simulink model "simuV6_restored_from_autosave"  (R2016a)
settings: Solver=VariableStepAuto  StartTime=0.0  StopTime=20  RelTol=1e-3
libraries: powerlib x15, powerlib_meascontrol x2, simulink x1
settings Model: Creator=EEE  LastModifiedBy=mbonea godwin

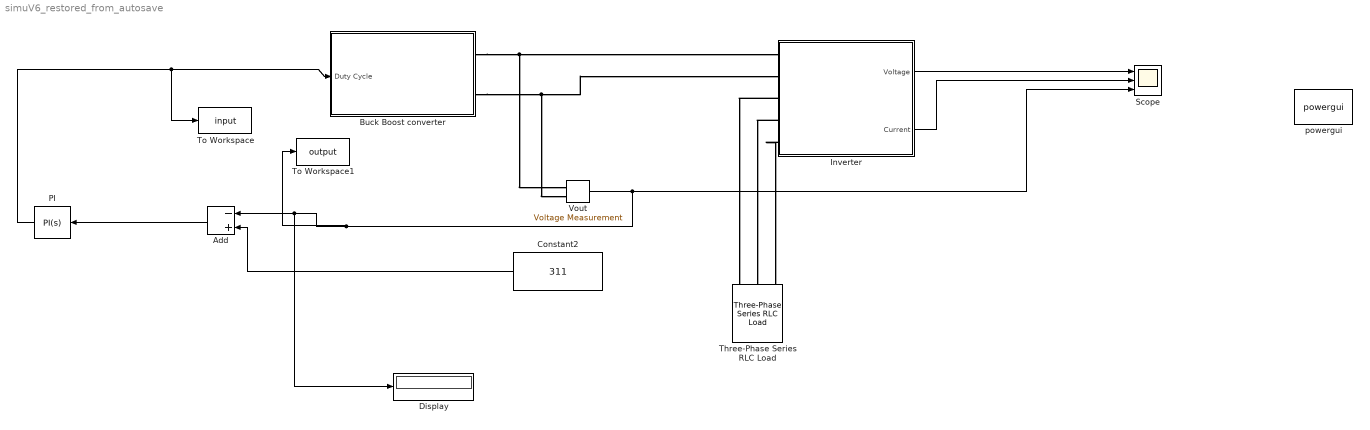
== system simuV6_restored_from_autosave ==
  Add : Sum  Inputs=-+
  Buck Boost converter : Subsystem
  Constant2 : Constant  Value=311
  Display : Display
  Inverter : Subsystem
  PI : simulink/Continuous/PID Controller  Controller=PI  TimeDomain=Continuous-time  SampleTime=-1  IntegratorMethod=Forward Euler  FilterMethod=Forward Euler  Form=Parallel  UseFilter=on  ControllerParametersSource=internal  P=43.0737287073608  I=6.97946285462644  D=0  N=100  InitialConditionSource=internal  InitialConditionForIntegrator=0  InitialConditionForFilter=0  ExternalReset=none  LimitOutput=on  UpperSaturationLimit=0.9  LowerSaturationLimit=0.1  LinearizeAsGain=on  AntiWindupMode=none  Kb=1  TrackingMode=off  Kt=1  PParamMin=[]  PParamMax=[]  IParamMin=[]  IParamMax=[]  DParamMin=[]  DParamMax=[]  NParamMin=[]  NParamMax=[]  KbParamMin=[]  KbParamMax=[]  KtParamMin=[]  KtParamMax=[]  POutMin=[]  POutMax=[]  IOutMin=[]  IOutMax=[]  DOutMin=[]  DOutMax=[]  NOutMin=[]  NOutMax=[]  KbOutMin=[]  KbOutMax=[]  KtOutMin=[]  KtOutMax=[]  IntegratorOutMin=[]  IntegratorOutMax=[]  FilterOutMin=[]  FilterOutMax=[]  SumOutMin=[]  SumOutMax=[]  SumI1OutMin=[]  SumI1OutMax=[]  SumI2OutMin=[]  SumI2OutMax=[]  SumI3OutMin=[]  SumI3OutMax=[]  SumDOutMin=[]  SumDOutMax=[]  SaturationOutMin=[]  SaturationOutMax=[]  IntegratorContinuousStateAttributes=''  IntegratorStateMustResolveToSignalObject=off  IntegratorRTWStateStorageClass=Auto  FilterContinuousStateAttributes=''  FilterStateMustResolveToSignalObject=off  FilterRTWStateStorageClass=Auto  DifferentiatorICPrevScaledInput=0  DifferentiatorOutMin=[]  DifferentiatorOutMax=[]
  Scope : Scope  NumInputPorts=3
  Three-Phase Series RLC Load : powerlib/Elements/Three-Phase Series RLC Load  LConnTagsString=A|B|C  Configuration=Y (grounded)  NominalVoltage=220  Vabc=[1e3 1e3 1e3]  Vabcp=[1e3 1e3 1e3]  NominalFrequency=50  UnbalancedPower=off  ActivePower=10e3  InductivePower=0  CapacitivePower=0  Pabc=[10e3 9e3 11e3]  QLabc=[100 90 110]  QCabc=[100 90 110]  Pabcp=[10e3 9e3 11e3]  QLabcp=[100 90 110]  QCabcp=[100 90 110]  Measurements=None  LoadType=constant Z
  To Workspace : ToWorkspace  VariableName=input  SaveFormat=Timeseries  SampleTime=-1
  To Workspace1 : ToWorkspace  VariableName=output  SaveFormat=Timeseries  SampleTime=-1
  Vout : powerlib/Measurements/Voltage Measurement  PhasorSimulation=off  OutputType=Complex  PSBequivalent=0
  powergui : powerlib/powergui  Priority=1  SimulationMode=Continuous  SolverType=Tustin/Backward Euler (TBE)  SampleTime=50e-6  frequency=60  SPID=on  DisableSnubberDevices=off  DisableRonSwitches=off  DisableVfSwitches=off  SwTol=0  DisplayEquations=off  Interpol=off  ExternalGateDelay=off  methode=off  Ts=10  FunctionMessages=off  echomessages=off  HookPort=off  EnableUseOfTLC=off  x0status=blocks  frequencyindice=0  Pbase=100e6  ErrMax=1e-4  Iterations=50  UnitsV=kV  UnitsW=MW  buscounter=0  RestoreLinks=warning  ResistiveCurrentMeasurement=off  Frange=[0:2:500]  Ylog=off  Xlog=on  ShowGrid=off  save=off  variable=ZData  structure=0  ZoomFFT=off  StartTime=0.0  cycles=1  DisplayStyle=1  fundamental=60  FreqAxis=off  MaxFrequency=1000  frequencyindicesteady=1  RmsSteady=1  display=off
  wires:
  Vout/1 -> To Workspace1/1, Display/1, Add/1, Scope/3
  Inverter/2(Current) -> Scope/2
  Inverter/1(Voltage) -> Scope/1
  Constant2/1 -> Add/2
  Add/1 -> PI/1
  PI/1 -> To Workspace/1, Buck Boost converter/1(Duty Cycle)
  connections:
  Buck Boost converter/RConn1 -- Vout/LConn1 -- Inverter/LConn1
  Buck Boost converter/RConn2 -- Vout/LConn2 -- Inverter/LConn2
  Inverter/LConn5 -- Three-Phase Series RLC Load/LConn3
  Inverter/LConn4 -- Three-Phase Series RLC Load/LConn2
  Inverter/LConn3 -- Three-Phase Series RLC Load/LConn1

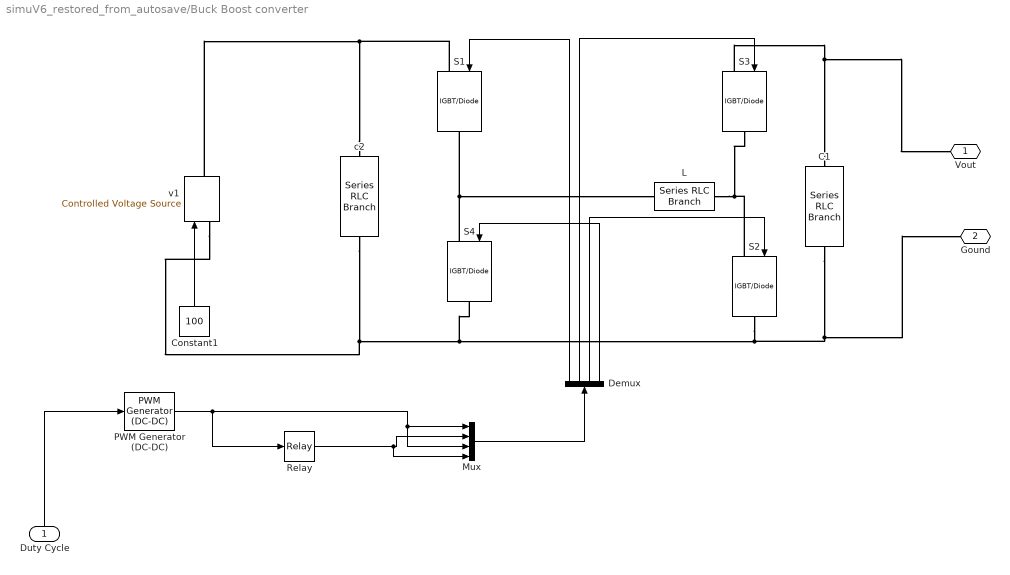
== system simuV6_restored_from_autosave/Buck Boost converter ==
  Duty Cycle : Inport
  "C1 " : powerlib/Elements/Series RLC Branch  LConnTagsString=__new0  RConnTagsString=__new0  BranchType=C  Resistance=1  Inductance=1e-3  SetiL0=off  InitialCurrent=0  Capacitance=20000000e-6  Setx0=off  InitialVoltage=0  Measurements=None
  Constant1 : Constant  Value=100
  Demux : Demux
  "L " : powerlib/Elements/Series RLC Branch  LConnTagsString=__new0  RConnTagsString=__new0  BranchType=L  Resistance=1  Inductance=1e-4  SetiL0=off  InitialCurrent=0  Capacitance=20000e-6  Setx0=off  InitialVoltage=0  Measurements=Branch voltage and current
  Mux : Mux
  PWM Generator (DC-DC) : powerlib_meascontrol/Pulse & Signal Generators/PWM Generator (DC-DC)  Fsw=5000  Ts=0
  Relay : Relay  OnOutputValue=0  OffOutputValue=1
  S{1..4} (4 alike) : powerlib/Power Electronics/IGBT//Diode  Ron=1e-3  Rs=1e5  Cs=inf  Measurements=off
  "c2 " : powerlib/Elements/Series RLC Branch  LConnTagsString=__new0  RConnTagsString=__new0  BranchType=RC  Resistance=10  Inductance=1e-3  SetiL0=off  InitialCurrent=0  Capacitance=15000e-6  Setx0=off  InitialVoltage=0  Measurements=None
  "v1 " : powerlib/Electrical Sources/Controlled Voltage Source  Initialize=on  Source_Type=DC  Amplitude=0  Phase=0  Frequency=0  Measurements=None
  Vout : PMIOPort  Port=1  Side=Right
  Gound : PMIOPort  Port=2  Side=Right
  wires:
  Duty Cycle/1 -> PWM Generator (DC-DC)/1
  Demux/2 -> S3/1
  Mux/1 -> Demux/1
  Demux/3 -> S2/1
  PWM Generator (DC-DC)/1 -> Relay/1, Mux/3, Mux/1
  Demux/4 -> S4/1
  Relay/1 -> Mux/4, Mux/2
  Constant1/1 -> "v1 "/1
  Demux/1 -> S1/1
  connections:
  S3/RConn1 -- "L "/LConn1 -- S2/LConn1
  S1/RConn1 -- "L "/RConn1 -- S4/LConn1
  S2/RConn1 -- Gound/RConn1 -- "C1 "/RConn1 -- S4/RConn1 -- "c2 "/RConn1 -- "v1 "/LConn1
  S3/LConn1 -- Vout/RConn1 -- "C1 "/LConn1
  "c2 "/LConn1 -- "v1 "/RConn1 -- S1/LConn1

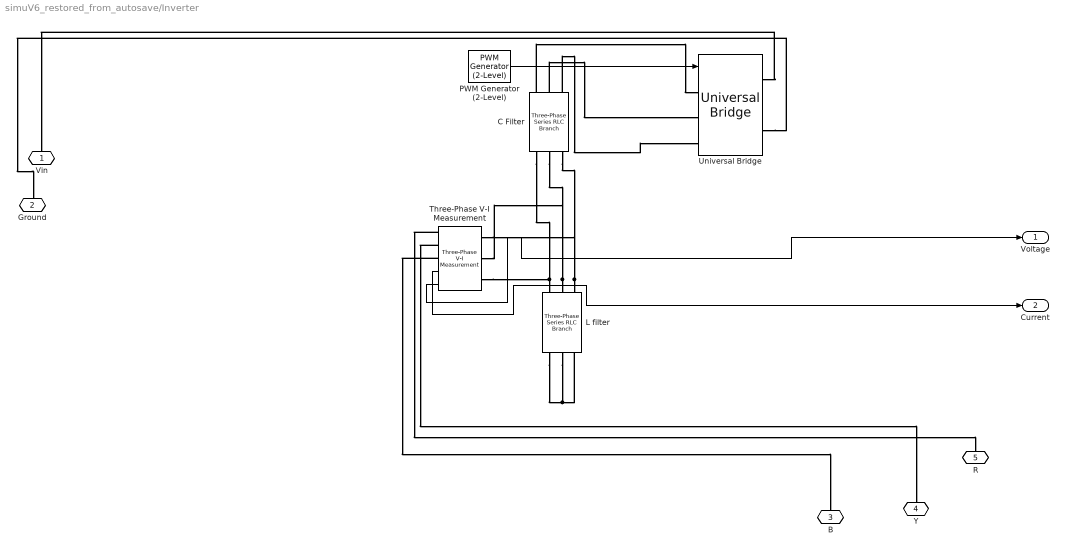
== system simuV6_restored_from_autosave/Inverter ==
  C Filter : powerlib/Elements/Three-Phase Series RLC Branch  LConnTagsString=A|B|C  RConnTagsString=A|B|C  BranchType=L  Resistance=1  Inductance=2.97e-3  Capacitance=2.97e-3  Measurements=None
  L filter : powerlib/Elements/Three-Phase Series RLC Branch  LConnTagsString=A|B|C  RConnTagsString=A|B|C  BranchType=C  Resistance=1  Inductance=2.97e-3  Capacitance=5.33e-5  Measurements=None
  PWM Generator (2-Level) : powerlib_meascontrol/Pulse & Signal Generators/PWM Generator (2-Level)  ModulatorType=Three-phase bridge (6 pulses)  ModulatorMode=Unsynchronized  Fc=27*50*3  Pc=90  nF=27  MinMax=[ -1 1 ]  SamplingTechnique=Natural  ModulatingSignals=on  m=0.8  Freq=50  Phase=0  Ts=0  ShowCarrierOutport=off
  Three-Phase V-I Measurement : powerlib/Measurements/Three-Phase V-I Measurement  VoltageMeasurement=phase-to-ground  SetLabelV=off  LabelV=Vabc  Vpu=off  VpuLL=off  CurrentMeasurement=yes  SetLabelI=off  LabelI=Iabc  Ipu=off  Pbase=100e6  Vbase=500e3  OutputType=Complex  PhasorSimulation=off  PSBequivalent=0
  Universal Bridge : powerlib/Power Electronics/Universal Bridge  Arms=3  SnubberResistance=1e5  SnubberCapacitance=inf  Device=IGBT / Diodes  Ron=1e-3  Lon=0  ForwardVoltages="[  0  0  ]"  ForwardVoltage=0  GTOparameters=[ 10e-6 , 20e-6 ]  IGBTparameters=[ 1e-6 , 2e-6 ]  Measurements=None  Measurements_2=None  converterType=Rectifier
  Vin : PMIOPort  Port=1  Side=Left
  Ground : PMIOPort  Port=2  Side=Left
  B : PMIOPort  Port=3  Side=Left
  Y : PMIOPort  Port=4  Side=Left
  R : PMIOPort  Port=5  Side=Left
  Voltage : Outport
  Current : Outport  Port=2
  wires:
  Three-Phase V-I Measurement/2 -> Current/1
  Three-Phase V-I Measurement/1 -> Voltage/1
  PWM Generator (2-Level)/1 -> Universal Bridge/1
  connections:
  Universal Bridge/RConn2 -- Ground/RConn1
  L filter/LConn1 -- C Filter/RConn1 -- Three-Phase V-I Measurement/LConn1
  L filter/LConn2 -- C Filter/RConn2 -- Three-Phase V-I Measurement/LConn2
  L filter/LConn3 -- C Filter/RConn3 -- Three-Phase V-I Measurement/LConn3
  C Filter/LConn3 -- Universal Bridge/LConn3
  C Filter/LConn2 -- Universal Bridge/LConn2
  C Filter/LConn1 -- Universal Bridge/LConn1
  L filter/RConn1 -- L filter/RConn2 -- L filter/RConn3
  Three-Phase V-I Measurement/RConn2 -- Y/RConn1
  Three-Phase V-I Measurement/RConn1 -- B/RConn1
  Universal Bridge/RConn1 -- Vin/RConn1
  Three-Phase V-I Measurement/RConn3 -- R/RConn1
